simulink model "Threephase_power"  (R2021a)
settings: Solver=VariableStepAuto  StartTime=0.0  StopTime=10.0  RelTol=1e-3
settings Model: Creator=Davie  LastModifiedBy=Davie

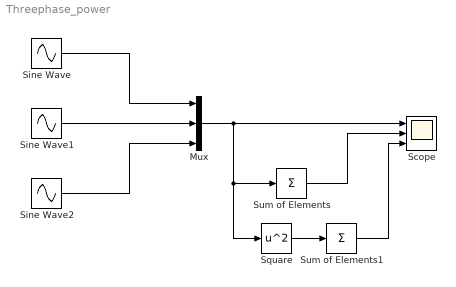
== system Threephase_power ==
  Mux : Mux  Inputs=3
  Scope : Scope  NumInputPorts=3
  Sine Wave : Sin  SampleTime=0
  Sine Wave1 : Sin  Phase=-120*pi/180  SampleTime=0
  Sine Wave2 : Sin  Phase=120*pi/180  SampleTime=0
  Square : Math  Operator=square  SaturateOnIntegerOverflow=on
  Sum of Elements : Sum  Inputs=+
  Sum of Elements1 : Sum  Inputs=+
  wires:
  Sine Wave1/1 -> Mux/2
  Mux/1 -> Square/1, Sum of Elements/1, Scope/1
  Sum of Elements/1 -> Scope/2
  Square/1 -> Sum of Elements1/1
  Sum of Elements1/1 -> Scope/3
  Sine Wave/1 -> Mux/1
  Sine Wave2/1 -> Mux/3
